simulink model "FULLsystem"  (R2024b)
settings: Solver=FixedStepAuto  StartTime=0.0  StopTime=inf  RelTol=1e-3
undefined symbols (not defined in the file or in its folder): QAM
libraries: commsync2 x2, commfilt2 x2, commdigbbndam3 x2, commchan3 x1, commrfcorlib x1
settings Model: Creator=J_mas  LastModifiedBy=J_mas

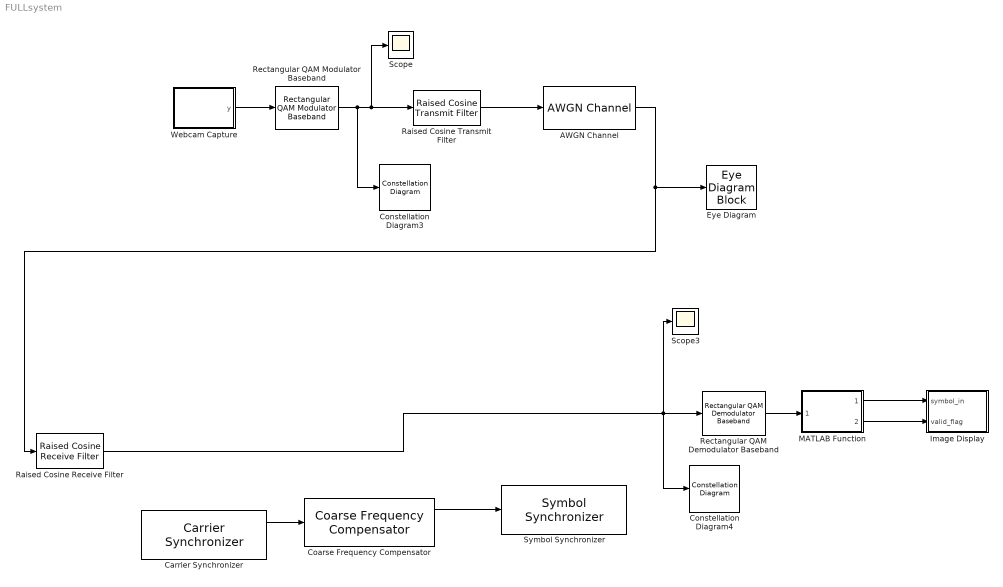
== system FULLsystem ==
  AWGN Channel : commchan3/AWGN Channel  LegacyMode=off  NoiseMethod="Signal to noise ratio  (SNR)"  noiseMode="Signal to noise ratio  (SNR)"  EbNo=10  EsNo=10  SNR=30  BitsPerSymbol=1  SignalPower=1  SamplesPerSymbol=1  SymbolPeriod=1  VarianceSource=Parameter  Variance=1  RandomStream=Global stream  Seed=67  SimulateUsing=Code generation
  Carrier Synchronizer : commsync2/Carrier Synchronizer  Modulation=QAM  ModulationPhaseOffset=Auto  CustomPhaseOffset=0  SamplesPerSymbol=8  DampingFactor=0.707  NormalizedLoopBandwidth=0.01  EstimatedPhaseErrorOutputPort=on  SimulateUsing=Code generation
  Coarse Frequency Compensator : commrfcorlib/Coarse Frequency Compensator  Modulation=QAM  Algorithm=FFT-based  FrequencyResolution=100  MaximumFrequencyOffset=5e3  SamplesPerSymbol=4  EstimatedFreqOffsetPort=on  SimulateUsing=Code generation
      settings: LibrarySourceBlock=|
      | commsync2/Coarse Frequency
      | Compensator
  Constellation Diagram3 : ConstellationDiagram  WindowPosition=[141.000000,91.000000,313.000000,260.000000,]  Visible=on  ScopeFrameLocation=window  SamplesPerSymbol=8  SymbolsToDisplaySource=Property  SymbolsToDisplay=100  ReferenceConstellation=64-QAM  XLimits=[-3.19,3.19]  YLimits=[-2.54,2.54]
  Constellation Diagram4 : ConstellationDiagram  WindowPosition=[885.000000,105.000000,303.000000,272.000000,]  Visible=on  ScopeFrameLocation=window  SamplesPerSymbol=8  SymbolsToDisplaySource=Property  SymbolsToDisplay=100  ReferenceConstellation=64-QAM  XLimits=[-3.19,3.19]  YLimits=[-2.54,2.54]
  Eye Diagram : EyeDiagramBlock  WindowPosition=[49.000000,-13.000000,800.000000,500.000000,]  Visible=on  ScopeFrameLocation=window  YLimits=[-3.4421337861281915,3.9515401682071]
  Image Display : MATLAB Function  TreatAsAtomicUnit=on
  MATLAB Function : MATLAB Function  TreatAsAtomicUnit=on
  Raised Cosine Receive Filter : commfilt2/Raised Cosine Receive Filter  filtType=Square root  R=0.2  filtSpan=10  N=8  downFactor=8  downOffset=0  filterGain=1  InputProcessing=Columns as channels (frame based)  RateOptions=Enforce single-rate processing  framing=Mute  checkCoeff=off  variableName=rcRxFilt  currentFiltSpan=10  D=5  inputOffset=0  sampMode=Mute  saveAsFlag=0  rateMode=Downsampling  checkGain=Normalized  launchFVT=on  roundingMode=Floor  overflowMode=off  coeffDataTypeStr=Inherit: Same word length as input  coeffMin=[]  coeffMax=[]  coeffLastDataTypeStr=Inherit: Same word length as input  accumDataTypeStr=Inherit: Same as product output  accumLastDataTypeStr=Inherit: Same as product output  outputDataTypeStr=Inherit: Same as accumulator  outputMin=[]  outputMax=[]  outputLastDataTypeStr=Inherit: Same as accumulator
  Raised Cosine Transmit Filter : commfilt2/Raised Cosine Transmit Filter  filtType=Square root  R=0.2  filtSpan=10  N=8  filterGain=1  InputProcessing=Columns as channels (frame based)  RateOptions=Enforce single-rate processing  framing=Mute  checkCoeff=off  variableName=rcTxFilt  checkGain=Normalized  sampMode=Mute  saveAsFlag=0  currentFiltSpan=10  D=(10)/2  launchFVT=on  roundingMode=Floor  overflowMode=off  coeffDataTypeStr=Inherit: Same word length as input  coeffMin=[]  coeffMax=[]  coeffLastDataTypeStr=Inherit: Same word length as input  outputDataTypeStr=Inherit: Same as accumulator  outputMin=[]  outputMax=[]  outputLastDataTypeStr=Inherit: Same as accumulator
  Rectangular QAM Demodulator Baseband : commdigbbndam3/Rectangular QAM Demodulator Baseband  M=64  OutType=Integer  DecType=Hard decision  VarSource=Dialog  Variance=1  Dec=Gray  Mapping=[0:15]  PowType=Min. distance between symbols  MinDist=2  AvgPow=1  PeakPow=1  Ph=0  outDtype1=Inherit via internal rule  outDtype2=uint8  derotateFactorWordLen=16  derotateFactorDataTypeStr=Inherit: Same word length as input  derotateFactorLastDataTypeStr=Inherit: Same word length as input  denormFactorWordLen=16  denormFactorDataTypeStr=Inherit: Same word length as input  denormFactorLastDataTypeStr=Inherit: Same word length as input  prodOutWordLen=32  prodOutOverflowMode=Wrap  prodOutRoundingMode=Floor  prodOutOvFlMode=off  prodOutOvFlModeLastStrValue=off  sumWordLen=32
  Rectangular QAM Modulator Baseband : commdigbbndam3/Rectangular QAM Modulator Baseband  M=64  InType=Integer  Enc=Gray  Mapping=[0:15]  PowType=Min. distance between symbols  MinDist=2  AvgPow=1  PeakPow=1  Ph=0  outDtype=double  outWordLen=16  outUDDataType=sfix(16)  outFracLenMode=Best precision  outFracLen=15  outDataTypeStr=double  outLastDataTypeStr=double
  Scope : Scope
  Scope3 : Scope
  Symbol Synchronizer : commsync2/Symbol Synchronizer  Modulation=PAM/PSK/QAM  TimingErrorDetector=Zero-Crossing (decision-directed)  SamplesPerSymbol=8  DampingFactor=1  NormalizedLoopBandwidth=0.01  DetectorGain=2.7  TimingErrorOutputPort=on  SimulateUsing=Code generation
  Webcam Capture : MATLAB Function  TreatAsAtomicUnit=on  SystemSampleTime=1/40000
  wires:
  Rectangular QAM Modulator Baseband/1 -> Constellation Diagram3/1, Scope/1, Raised Cosine Transmit Filter/1
  Raised Cosine Transmit Filter/1 -> AWGN Channel/1
  Webcam Capture/1(y) -> Rectangular QAM Modulator Baseband/1
  AWGN Channel/1 -> Eye Diagram/1, Raised Cosine Receive Filter/1
  Raised Cosine Receive Filter/1 -> Constellation Diagram4/1, Scope3/1, Rectangular QAM Demodulator Baseband/1
  Carrier Synchronizer/1 -> Coarse Frequency Compensator/1
  Coarse Frequency Compensator/1 -> Symbol Synchronizer/1
  MATLAB Function/1(payload_symbol) -> Image Display/1(symbol_in)
  MATLAB Function/2(frame_valid) -> Image Display/2(valid_flag)
  Rectangular QAM Demodulator Baseband/1 -> MATLAB Function/1(demod_symbol)

== matlab function FULLsystem/Webcam Capture ==
  data: y output
function y = fcn() %#codegen
    coder.extrinsic('webcam', 'snapshot', 'imresize', 'rgb2gray', 'imshow', 'tic', 'toc', 'fprintf');
    
    persistent cam packetBuffer packetIndex initialized startTime symbolCount
    
    y = uint8(0); % Output type should match Modulator input (usually integer)
    
    % Barker code parameters
    BARKER_LENGTH = 13; % Length-13 Barker code for good autocorrelation
    IMG_ROWS = 320;
    IMG_COLS = 240;
    PAYLOAD_LENGTH = IMG_ROWS * IMG_COLS;

    PACKET_LENGTH = BARKER_LENGTH + PAYLOAD_LENGTH;
    
    if isempty(initialized)
        cam = webcam(1);
        startTime = tic;
        
        % Buffer now holds complete packets (preamble + payload)
        packetBuffer = uint8(zeros(PACKET_LENGTH, 1));
        packetIndex = PACKET_LENGTH + 1; % Start beyond buffer to trigger capture
        symbolCount = 0;
        initialized = true;
    end
    
    % When we've transmitted the entire packet, capture a new frame
    if packetIndex > PACKET_LENGTH
        % Capture and process webcam image
        rawImg = snapshot(cam);
        imgResized = imresize(rawImg, [IMG_ROWS, IMG_COLS]);
        imgGrayRaw = rgb2gray(imgResized);
        imshow(imgGrayRaw);
        
        imgGray = uint8(zeros(IMG_ROWS, IMG_COLS));
        imgGray = imgGrayRaw;
        
        % Flatten the image and convert to 6-bit symbols (0-63)
        temp = reshape(imgGray, PAYLOAD_LENGTH, 1);
        payload = uint8(floor(double(temp) / 4)); % Map 0-255 to 0-63
        
        % Create Barker code preamble
        % Standard 13-bit Barker: [1 1 1 1 1 -1 -1 1 1 -1 1 -1 1]
        % Map to 6-bit symbols: use 63 for '1' and 0 for '-1' for good separation
        barker_preamble = uint8([63 63 63 63 63 0 0 63 63 0 63 0 63]');
        
        % Construct packet: [Preamble | Payload]
        packetBuffer(1:BARKER_LENGTH) = barker_preamble;
        packetBuffer(BARKER_LENGTH+1:PACKET_LENGTH) = payload;
        
        % Reset index to start of packet
        packetIndex = 1;
        
        % Statistics
        elapsedTime = toc(startTime);
        symbolRate = symbolCount / elapsedTime;
        fprintf('Symbol Rate: %.2f symbols/sec\n', symbolRate);
        fprintf('Packet Rate: %.2f packets/sec\n', symbolCount / (PACKET_LENGTH * elapsedTime));
    end
    
    % Output one symbol per call
    if packetIndex <= PACKET_LENGTH
        y = packetBuffer(packetIndex);
        packetIndex = packetIndex + 1;
        symbolCount = symbolCount + 1;
    end
end

== matlab function FULLsystem/MATLAB Function ==
  data: demod_symbol input; payload_symbol output; frame_valid output
function [payload_symbol, frame_valid] = barkerFrameDetector(demod_symbol)
%#codegen

assert(isscalar(demod_symbol));

sym_in = uint8(demod_symbol);

payload_symbol = uint8(0);
frame_valid = false;

persistent preambleBuffer collecting payloadCounter

if isempty(collecting)
    preambleBuffer = zeros(13,1,'uint8');
    collecting = false;
    payloadCounter = uint32(0);
end

PREAMBLE = uint8([63;63;63;63;63;0;0;63;63;0;63;0;63]);
PAYLOAD_LIMIT = uint32(76800);

if ~collecting

    for i = 1:12
        preambleBuffer(i) = preambleBuffer(i+1);
    end
    preambleBuffer(13) = sym_in;

    matches = uint8(0);
    for i = 1:13
        if preambleBuffer(i) == PREAMBLE(i)
            matches = matches + 1;
        end
    end

    if matches >= 11
        collecting = true;
        payloadCounter = uint32(0);
    end

else

    payloadCounter = payloadCounter + 1;

    if payloadCounter <= PAYLOAD_LIMIT
        payload_symbol = sym_in;
        frame_valid = true;
    end

    if payloadCounter >= PAYLOAD_LIMIT
        collecting = false;
        payloadCounter = uint32(0);
    end

end

end

== matlab function FULLsystem/Image Display ==
  data: symbol_in input; valid_flag input
function reconstruct_image(symbol_in, valid_flag) %#codegen
    coder.extrinsic('imshow', 'figure', 'drawnow', 'title');
    
    persistent imgBuffer symbolCount fig initialized
    
    if isempty(initialized)
        IMG_ROWS = 320;
        IMG_COLS = 240;
        imgBuffer = uint8(zeros(IMG_ROWS, IMG_COLS));
        symbolCount = 0;
        fig = figure('Name', 'Received Image');
        initialized = true;
    end
    
    % Only accumulate if we have valid payload data
    if valid_flag
        symbolCount = symbolCount + 1;
        
        if symbolCount <= 76800
            imgBuffer(symbolCount) = symbol_in * 4;
        end
        
        % Display complete frame
        if symbolCount == 76800
            imshow(imgBuffer);
            title('Received Image');
            drawnow;
            
            % Reset for next frame
            symbolCount = 0;
        end
    end
end
